simulink model "Encapsulated_Odd_Deadzone_test"  (Simulink 7.3)
settings: Solver=ode45  StartTime=0.0  StopTime=10.0  RelTol=1e-3
settings Model: Creator=MD710  LastModifiedBy=MD710
settings DebuggingCC: SaveWithParameterizedLinksMsg=none  SolverPrmCheckMsg=none  MultiTaskDSMMsg=warning  MultiTaskCondExecSysMsg=none  FcnCallInpInsideContextMsg=Enable All  StrictBusMsg=None
settings HardwareCC: TargetHWDeviceType=32-bit Generic
settings RTWCC: IncludeERTFirstTime=on
settings GRTTargetCC: TargetFcnLib=ansi_tfl_tmw.mat

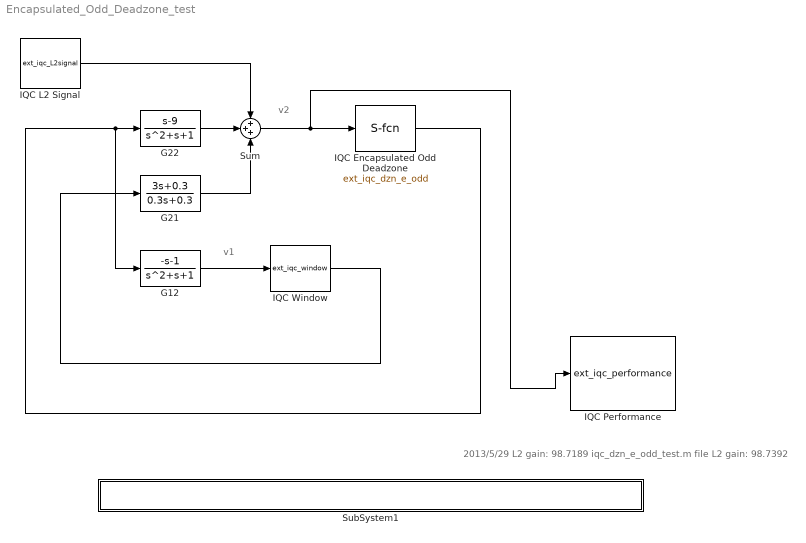
== system Encapsulated_Odd_Deadzone_test ==
  note: v2
  note: v1
  note: 2013/5/29 L2 gain: 98.7189
      | iqc_dzn_e_odd_test.m file L2 gain: 98.7392
  G12 : TransferFcn  Numerator=[-1 -1]  Denominator=[1 1 1]
  G21 : TransferFcn  Numerator=[3 0.3]  Denominator=[0.3 0.3]
  G22 : TransferFcn  Numerator=[1 -9]  Denominator=[1 1 1]
  IQC Encapsulated Odd Deadzone : M-S-Function  FunctionName=ext_iqc_dzn_e_odd  Parameters=pole,def_num_h,slo_bou,out_var  mask(IQC Encapsulated Odd Deadzone(ver:0.1)){pole=[1.8], def_num_h=0, slo_bou=0.3, out_var=''}
      mask prompts: pole "Pole:(Default: [1])"; def_num_h "Defines Number of Terms in Expansion for H:(Default: 0)"; slo_bou "Slope Bound for The Encapsulated Nonlinearity:(Default: 1)"; out_var "Output Variable:(Default: empty)"
      mask help:
      | Example: [w,h_0,H,F,xp,xm]=iqc_dzn_e_odd(v,a,N,kdzn)
      | Pole:
      |         [a]
      | Defines Number of Terms in Expansion for H:
      |          N
      | Slope Bound for The Encapsulated Nonlinearity:
      |         kdzn
      | Output Variable:
      |     {'h_0','H','F','xp','xm'}
      mask Help: eval('doc iqc_dzn_e_odd')
      mask Display: plot(0,0,100,100,[60,30,30,60,60],[90,90,60,60,90],[30,30,60,60,30],[40,10,10,40,40],[30,10,10,3,30],[25,25,76,76,76],[80,80,60],[72,25,25],[60,77],[76,76],[82,80,77,80,82,98],[76,72,76,80,76,76],[58,50,40,32],[88,76,76,63],[42,45,45,50],[15,17,34,36]);
  IQC L2 Signal : M-S-Function  FunctionName=ext_iqc_L2signal  Parameters=sig_size,sam_time,sig_type,tru_time,sig_amp,sig_fre,user_cus  mask(IQC L2 signal(ver:0.1)){sig_size=1, sam_time=0, sig_type=Step, tru_time=10, sig_amp=1, sig_fre=1, user_cus='2*exp(3*t)'}
      mask prompts: sig_size "Signal Dimension:(Default: 1)"; sam_time "Sample Time:(Default: 0)"; sig_type "Signal Type:"; tru_time "Truncation Time:"; sig_amp "Maximum Amplitude:"; sig_fre "Frequency:"; user_cus "Custom:"
      mask help:
      | Important:
      | In IQC procedure step (as commond iqc_gain_tbx, the task is get
      | L2 gain value), regardless of the user to choose which option (ex sine...),
      | here regarded as generalized L2 signal.
      mask StyleString: edit,edit,popup(Step|Square wave|Sine wave|Custom|Random|External),edit,edit,edit,edit
      mask CallbackString: ||iqc_block_cho(gcb,'L2signal_type')||||
      mask TabNameString: Generalized Parameters,Generalized Parameters,Simulink Parameters,Simulink Parameters,Simulink Parameters,Simulink Parameters,Simulink Parameters
      mask Display: plot(0:0.1:10,[sin(0:0.1:6.2) zeros(1,38)])
  IQC Performance : M-S-Function  FunctionName=ext_iqc_performance  Parameters=imp_met,save_lin_com,isiqcbode,fre_ran,uselmitool,lmi_par  mask(IQC Performance(ver:0.1)){imp_met=Only Calculation, save_lin_com=off, isiqcbode=off, fre_ran='', uselmitool=lmilab, lmi_par=''}
      mask prompts: imp_met "Implementation Methods"; save_lin_com "Save the Linear File and Command File"; isiqcbode "Display IQC Bode Figure"; fre_ran "Frequency Range:(Default: empty)"; uselmitool "LMI Tool:"; lmi_par "Parameter:(if empty use define)"
      mask help:
      | Important:
      | In IQC toolbox calculate step (as commond iqc_gain_tbx, the task is get
      | L2 gain value), regardless of the user to connect any signal input(Even if
      | not a signal), here regarded as generalized L2 signal.
      |
      | Example 1: setlmioptions('',[0 200 0 0 777])
      | the block parameter is
      | LMI Tool: lmilab
      | Parameter:
      |        [0 200 0 0 777]
      |
      | Example 2: setlmioptions('yalmip','solver','sdpt3','verbose',1)
      | the block parameter is
      | LMI Tool: yalmip
      | Parameter:
      |        {'solver',sdpt3','verbose',1}
      mask Help:
      | <a href="matlab:doc abst_init_iqc;">abst_init_iqc</a>
      | <a href="matlab:doc setlmioptions;">setlmioptions</a>
      | <a href="matlab:doc iqc_gain_tbx;">iqc_gain_tbx</a>
      mask StyleString: popup(Calculation and Simulation|Only Calculation|Only Simulation),checkbox,checkbox,edit,popup(lmilab|yalmip),edit
      mask CallbackString: iqc_block_cho(gcb,'performance_imp')||iqc_block_cho(gcb,'performance_bodefre')|||
      mask TabNameString: Parameter,Parameter,Parameter,Parameter,LMI Parameter,LMI Parameter
      mask Display: fprintf('In -> Out \n performance \n L2 gain:\n%4.4f',98.7189);
  IQC Window : M-S-Function  FunctionName=ext_iqc_window  Parameters=max_del,pole,out_var  mask(IQC Window(ver:0.1)){max_del=0.27, pole=[], out_var=''}
      mask prompts: max_del "Maximum Time Delay:(Default: 1)"; pole "Pole:(Default: [])"; out_var "Output Variable:(Default: empty)"
      mask help:
      | Example: [w,X,Y]=iqc_window(v,T,a)
      | Maximum Time Delay:
      |            T
      | Pole:
      |           [a]
      | Output Variable:
      |          {'X','Y'}
      mask Help: eval('doc iqc_window')
      mask Display: plot(0,0,100,100,[84,94,4],[27,25,25],[94,84],[25,22],[15,15],[5,97],[12,15],[86,97],[18,15],[86,97],[81,70,70,16,16,6],[26,26,72,72,26,26],[71,71,15],[26,73,73]);
  SubSystem1 : Subsystem  mask{filename=iqc_dzn_e_odd_test.m}
      mask init:
      | x_dir=which(filename);
      | x=x_dir;
      settings: OpenFcn=|
      | x_dir=which('iqc_dzn_e_odd_test.m');
      | x=x_dir;
      | edit(x);
      mask Display: disp(['MATLAB file: ' x]);
  Sum : Sum  Inputs=+++
  wires:
  G22/1 -> Sum/2
  G21/1 -> Sum/3
  IQC L2 Signal/1 -> Sum/1
  G12/1 -> IQC Window/1
  IQC Window/1 -> G21/1
  Sum/1 -> IQC Performance/1, IQC Encapsulated Odd Deadzone/1
  IQC Encapsulated Odd Deadzone/1 -> G22/1, G12/1

== system Encapsulated_Odd_Deadzone_test/SubSystem1 ==
